simulink library "FUSA_EM_EMFL"  (R2023b)
settings: Solver=VariableStepAuto  StartTime=0.0  StopTime=10.0  RelTol=1e-3
undefined symbols (not defined in the file): FUSA_EM_EMFL_p1_TempMotDertCoefFrLe_na, FUSA_EM_EMFL_px_TempMotFrLeLkp_degC
libraries: simulink x1
settings Model: Creator=blatak  LastModifiedBy=blatak

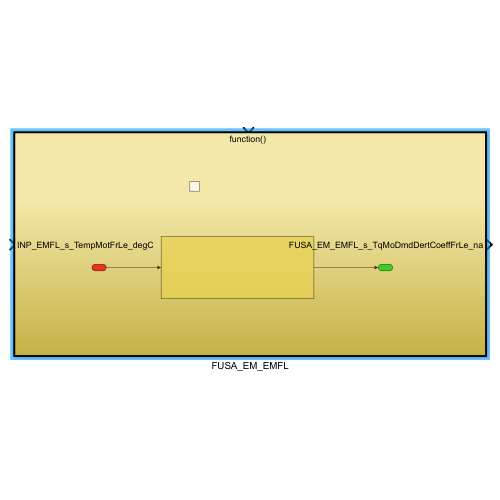
[thumbnail: Simulink's stored preview of the top-level diagram]
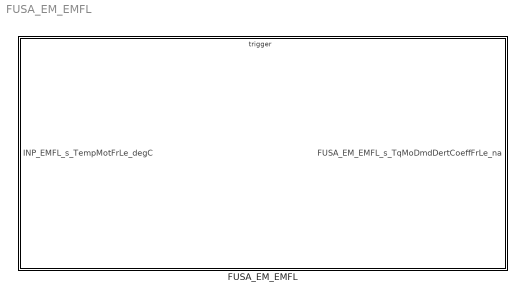
== system FUSA_EM_EMFL ==
  FUSA_EM_EMFL : Subsystem  TreatAsAtomicUnit=on

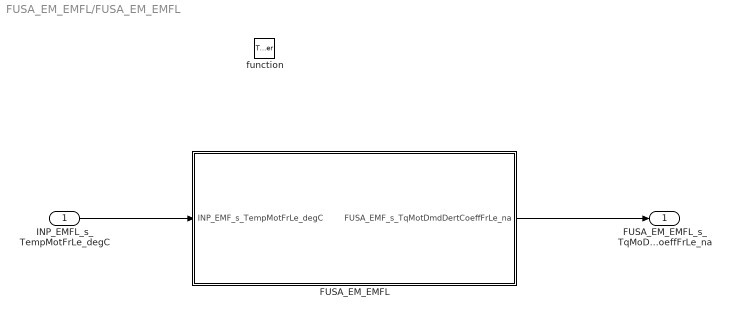
== system FUSA_EM_EMFL/FUSA_EM_EMFL ==
  INP_EMFL_s_TempMotFrLe_degC : Inport
  function : TriggerPort  TriggerType=function-call  VariantControl=(inherit)
  FUSA_EM_EMFL : Subsystem
  FUSA_EM_EMFL_s_TqMoDmdDertCoeffFrLe_na : Outport
  wires:
  INP_EMFL_s_TempMotFrLe_degC/1 -> FUSA_EM_EMFL/1(INP_EMF_s_TempMotFrLe_degC)
  FUSA_EM_EMFL/1(FUSA_EMF_s_TqMotDmdDertCoeffFrLe_na) -> FUSA_EM_EMFL_s_TqMoDmdDertCoeffFrLe_na/1

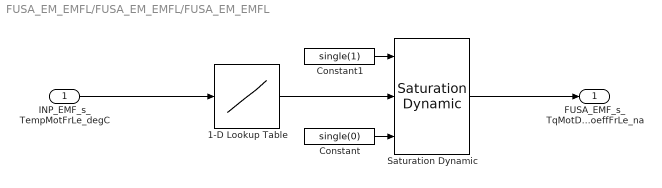
== system FUSA_EM_EMFL/FUSA_EM_EMFL/FUSA_EM_EMFL ==
  INP_EMF_s_TempMotFrLe_degC : Inport
  1-D Lookup Table : Lookup_n-D  NumberOfTableDimensions=1  BreakpointsForDimension1=FUSA_EM_EMFL_px_TempMotFrLeLkp_degC  Table=FUSA_EM_EMFL_p1_TempMotDertCoefFrLe_na  InternalRulePriority=Speed  RndMeth=Simplest
  Constant : Constant  Value=single(0)
  Constant1 : Constant  Value=single(1)
  Saturation Dynamic : simulink/Discontinuities/Saturation Dynamic  OutMin=[]  OutMax=[]  OutDataTypeStr=Inherit: Same as second input  OutDataType=fixdt(1, 16)  OutScaling=2^-10  DoSatur=off
  FUSA_EMF_s_TqMotDmdDertCoeffFrLe_na : Outport  Description=Derate torque coefficient front
  wires:
  Constant/1 -> Saturation Dynamic/3
  1-D Lookup Table/1 -> Saturation Dynamic/2
  Saturation Dynamic/1 -> FUSA_EMF_s_TqMotDmdDertCoeffFrLe_na/1
  INP_EMF_s_TempMotFrLe_degC/1 -> 1-D Lookup Table/1
  Constant1/1 -> Saturation Dynamic/1
